simulink model "CellModel_secOrd"  (R2016a)
settings: Solver=ode45  StartTime=0.0  StopTime=Tend  FixedStep=0.1  RelTol=1e-3
values from neighbouring files (symbols this model uses):
  beta1 = 1/(R1*C1)    (= 0.2)    [RCID_cal.m]    (also in errFun_multi.m = 1/(R1*C1))
  beta2 = 1/(R2*C2)    (= 0.5)    [RCID_cal.m]    (also in errFun_multi.m = 1/(R2*C2))
  capacity = cell_cap    [RCID_cal.m]    (also in errFun_multi.m)
  e0 = V_OCV    [RCID_cal.m]    (also in errFun_multi.m)
  gamma1 = 1/C1    (= 0.0005)    [RCID_cal.m]    (also in errFun_multi.m = 1/C1)
  gamma2 = 1/C2    (= 0.001)    [RCID_cal.m]    (also in errFun_multi.m = 1/C2)
  initialSoC = interp1(e0,s0,V_data(1))    [RCID_cal.m]    (also in errFun_multi.m = interp1(e0_un,s0(ind_un),V_data(1)))
  r0 = opt_val(1)    [RCID_cal.m]    (also in errFun_multi.m = x(1))
settings Model: Creator=BJ  LastModifiedBy=Polina Brodsky
settings DataIOCC: LimitDataPoints=on  SaveFormat=Array  SignalLoggingSaveFormat=ModelDataLogs
settings OptimizationCC: ExpressionDepthLimit=2147483647
settings DebuggingCC: UnderspecifiedInitializationDetection=Classic  MergeDetectMultiDrivingBlocksExec=none  SolverPrmCheckMsg=warning  FcnCallInpInsideContextMsg=EnableAllAsWarning  StateNameClashWarn=warning
settings HardwareCC: ProdBitPerPointer=32  ProdLargestAtomicFloat=None  ProdIntDivRoundTo=Undefined  ProdEndianess=Unspecified  ProdWordSize=32  ProdHWDeviceType=32-bit Generic
settings ModelReferenceCC: PropagateSignalLabelsOutOfModel=off
settings ConfigComp: CovModelRefEnable=Off  CovSFcnEnable=off

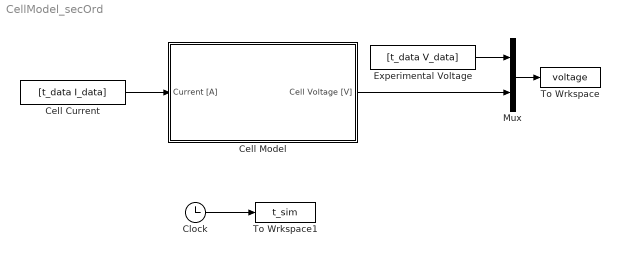
== system CellModel_secOrd ==
  Cell Current : FromWorkspace  VariableName=[t_data I_data]  SampleTime=0
  Cell Model : Subsystem
  Clock : Clock
  Experimental Voltage : FromWorkspace  VariableName=[t_data V_data]  SampleTime=0
  Mux : Mux  Inputs=2
  To Wrkspace : ToWorkspace  VariableName=voltage  SampleTime=-1
  To Wrkspace1 : ToWorkspace  VariableName=t_sim  SampleTime=-1
  wires:
  Cell Current/1 -> Cell Model/1(Current [A])
  Experimental Voltage/1 -> Mux/1
  Cell Model/1(" Cell Voltage [V]") -> Mux/2
  Mux/1 -> To Wrkspace/1
  Clock/1 -> To Wrkspace1/1

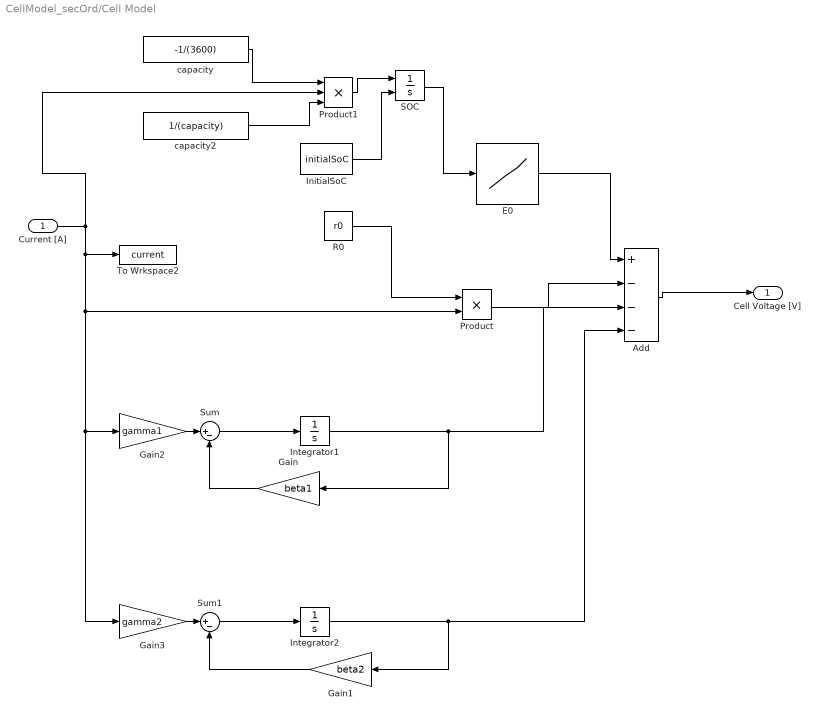
== system CellModel_secOrd/Cell Model ==
  Current [A] : Inport
  Add : Sum  Inputs=+---
  E0 : Lookup_n-D  NumberOfTableDimensions=1  BreakpointsForDimension1=linspace(0,1, length(e0))  Table=e0  RndMeth=Simplest  InputSameDT=on
  Gain : Gain  Gain=beta1
  Gain1 : Gain  Gain=beta2
  Gain2 : Gain  Gain=gamma1
  Gain3 : Gain  Gain=gamma2
  InitialSoC : Constant  Value=initialSoC
  Integrator1 : Integrator
  Integrator2 : Integrator
  Product : Product  RndMeth=Zero
  Product1 : Product  Inputs=3  RndMeth=Zero
  R0 : Constant  Value=r0
  SOC : Integrator  InitialConditionSource=external  InitialCondition=1
  Sum : Sum  Inputs=|+-
  Sum1 : Sum  Inputs=|+-
  To Wrkspace2 : ToWorkspace  VariableName=current  SampleTime=-1
  capacity : Constant  Value=-1/(3600)
  capacity2 : Constant  Value=1/(capacity)
  " Cell Voltage [V]" : Outport
  wires:
  InitialSoC/1 -> SOC/2
  capacity2/1 -> Product1/3
  E0/1 -> Add/1
  R0/1 -> Product/1
  Product/1 -> Add/2
  Add/1 -> " Cell Voltage [V]"/1
  capacity/1 -> Product1/1
  Product1/1 -> SOC/1
  Gain2/1 -> Sum/1
  Integrator1/1 -> Gain/1, Add/3
  Sum/1 -> Integrator1/1
  SOC/1 -> E0/1
  Gain/1 -> Sum/2
  Current [A]/1 -> Product1/2, To Wrkspace2/1, Product/2, Gain3/1, Gain2/1
  Gain3/1 -> Sum1/1
  Integrator2/1 -> Add/4, Gain1/1
  Sum1/1 -> Integrator2/1
  Gain1/1 -> Sum1/2
